simulink model "chap1_3n"  (Simulink 8.8)
settings: Solver=VariableStepAuto  StartTime=0.0  StopTime=10.0  RelTol=1e-3
settings Model: SuppressorTable=22 serialization::archive 11 0 3 0 0 0 0 0  Creator=guoshaopan  LastModifiedBy=guoshaopan
settings DataIOCC: LimitDataPoints=off  SaveFormat=Dataset  SignalLoggingSaveFormat=Dataset
settings OptimizationCC: LifeSpan=auto
settings DebuggingCC: UnderspecifiedInitializationDetection=Simplified  MergeDetectMultiDrivingBlocksExec=error  FcnCallInpInsideContextMsg=error  StateNameClashWarn=none  SFUnexpectedBacktrackingDiag=error  SFNoUnconditionalDefaultTransitionDiag=error  SFExecutionAtInitializationDiag=warning
settings HardwareCC: ProdBitPerPointer=64  ProdBitPerSizeT=64  ProdBitPerPtrDiffT=64  ProdLargestAtomicFloat=Float  ProdIntDivRoundTo=Zero  ProdEndianess=LittleEndian  ProdWordSize=64  ProdHWDeviceType=Intel->x86-64 (Windows64)
settings ModelReferenceCC: PropagateSignalLabelsOutOfModel=on
settings GRTTargetCC: TargetLangStandard=C99 (ISO)  GeneratePreprocessorConditionals=Use local settings  CombineOutputUpdateFcns=on  GRTInterface=off
settings ConfigComp: CovMetricSettings=dwe  CovHtmlReporting=off  CovSaveCumulativeToWorkspaceVar=off  CovSaveSingleToWorkspaceVar=off  CovExternalEMLEnable=on

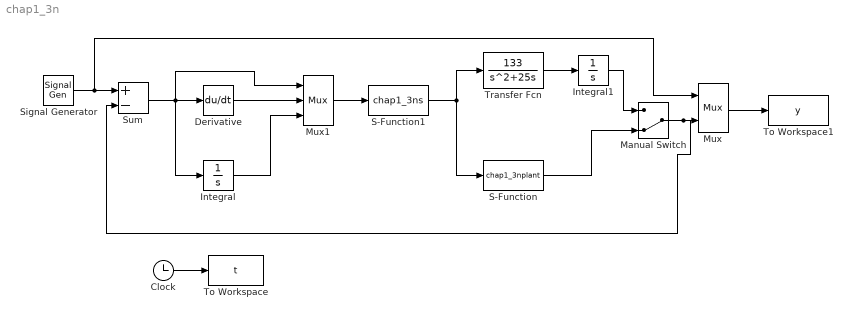
== system chap1_3n ==
  Clock : Clock
  Derivative : Derivative
  Integral : Integrator
  Integral1 : Integrator
  Manual Switch : ManualSwitch  CurrentSetting=0
  Mux : Mux  Inputs=2
  Mux1 : Mux  Inputs=3
  S-Function : S-Function  FunctionName=chap1_3nplant  SFunctionDeploymentMode=off  EnableBusSupport=off
  S-Function1 : S-Function  FunctionName=chap1_3ns  SFunctionDeploymentMode=off  EnableBusSupport=off
  Signal Generator : SignalGenerator  Frequency=0.20
  Sum : Sum  Inputs=+-
  "To Workspace " : ToWorkspace  VariableName=t  SampleTime=-1
  To Workspace1 : ToWorkspace  VariableName=y  SampleTime=-1
  Transfer Fcn : TransferFcn  Numerator=[133]  Denominator=[1 25 0]
  wires:
  Signal Generator/1 -> Mux/1, Sum/1
  Sum/1 -> Mux1/1, Integral/1, Derivative/1
  Derivative/1 -> Mux1/2
  Mux1/1 -> S-Function1/1
  S-Function1/1 -> S-Function/1, Transfer Fcn/1
  Transfer Fcn/1 -> Integral1/1
  Integral1/1 -> Manual Switch/1
  S-Function/1 -> Manual Switch/2
  Mux/1 -> To Workspace1/1
  Manual Switch/1 -> Sum/2, Mux/2
  Clock/1 -> "To Workspace "/1
  Integral/1 -> Mux1/3
